simulink model "EulerRatesFromAngularVelocity"  (R2016a)
settings: Solver=VariableStepAuto  SolverMode=SingleTasking  StartTime=0.0  StopTime=10.0  RelTol=1e-3
settings Model: Creator=Alireza  LastModifiedBy=Alireza
settings DataIOCC: ReturnWorkspaceOutputs=on
settings DebuggingCC: SFUnexpectedBacktrackingDiag=error  SFNoUnconditionalDefaultTransitionDiag=error
settings SFSimCC: SimUseLocalCustomCode=on
settings RTWCC: RTWUseLocalCustomCode=on
settings GRTTargetCC: TargetLangStandard=C99 (ISO)
settings ConfigComp: CovMetricSettings=dwe  CovHtmlReporting=off  CovSaveCumulativeToWorkspaceVar=off  CovSaveSingleToWorkspaceVar=off  CovExternalEMLEnable=on

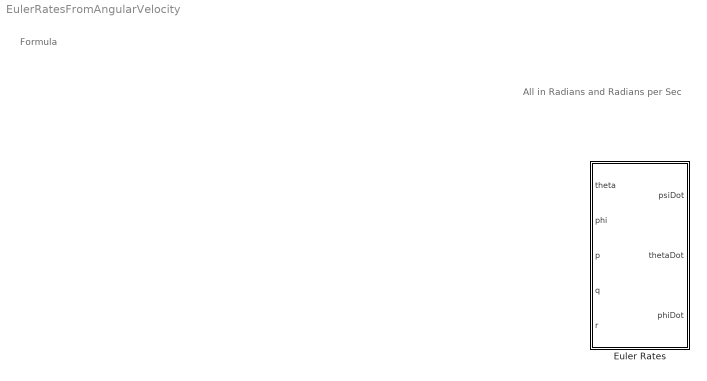
== system EulerRatesFromAngularVelocity ==
  note: Formula
  note: All in Radians and Radians per Sec
  Euler Rates : Subsystem

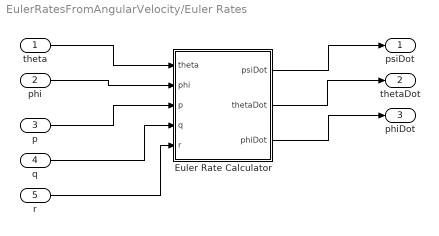
== system EulerRatesFromAngularVelocity/Euler Rates ==
  theta : Inport
  phi : Inport  Port=2
  p : Inport  Port=3
  q : Inport  Port=4
  r : Inport  Port=5
  Euler Rate Calculator : MATLAB Function  TreatAsAtomicUnit=on
  psiDot : Outport
  thetaDot : Outport  Port=2
  phiDot : Outport  Port=3
  wires:
  phi/1 -> Euler Rate Calculator/2(phi)
  theta/1 -> Euler Rate Calculator/1(theta)
  p/1 -> Euler Rate Calculator/3(p)
  q/1 -> Euler Rate Calculator/4(q)
  r/1 -> Euler Rate Calculator/5(r)
  Euler Rate Calculator/1(psiDot) -> psiDot/1
  Euler Rate Calculator/2(thetaDot) -> thetaDot/1
  Euler Rate Calculator/3(phiDot) -> phiDot/1

== matlab function EulerRatesFromAngularVelocity/Euler Rates/Euler Rate Calculator ==
  data: theta input; psiDot output; phi input; p input; q input; r input; thetaDot output; phiDot output
function [psiDot,thetaDot,phiDot] = fcn(theta,phi,p,q,r)

psiDot =  sin(phi)/cos(theta)*q + cos(phi)/cos(theta)*r;
thetaDot = cos(phi)*q - sin(phi)*r;
phiDot = p + sin(phi)*tan(theta)*q + cos(phi)*tan(theta)*r;
end
